simulink model "FinalSimuLab6"  (R2018b)
settings: Solver=VariableStepAuto  StartTime=0.0  StopTime=100.0  RelTol=1e-3
values from neighbouring files (symbols this model uses):
  A1 = k1    (= 8)    [FinalLab6.m]    (also in lab6.m = 2)
  a1 = Aw1*sqrt(2*g*h1max)/h1max    [FinalLab6.m]    (also in lab6.m = Aw1*sqrt(2*g*hm1)/hm1)
  A2 = k1    (= 8)    [FinalLab6.m]    (also in lab6.m = 2)
  a2 = Aw2*sqrt(2*g*h2max)/h2max    [FinalLab6.m]    (also in lab6.m = Aw2*sqrt(2*g*hm2)/hm2)
  dfwe1 = 0.1 * fwe1max    [FinalLab6.m]
  dt = 20    [FinalLab6.m]    (also in lab6.m = 10)
  fwe1 = fwe10(i)    [FinalLab6.m]    (also in lab6.m)
  fwe2 = 0    [FinalLab6.m]    (also in lab6.m)
  h10 = (fwe1 / a1) + h20    [FinalLab6.m]    (also in lab6.m = (fwe1+a1*h20)/a1)
  h20 = (fwe1 + fwe2)/a2    [FinalLab6.m]    (also in lab6.m = (fwe2+fwe1)/a2)
settings Model: Creator=wojciechkonury  LastModifiedBy=wojciechkonury

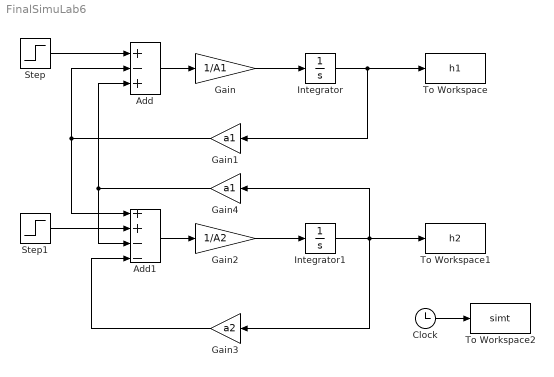
== system FinalSimuLab6 ==
  Add : Sum  Inputs=+-+
  Add1 : Sum  Inputs=++--
  Clock : Clock
  Gain : Gain  Gain=1/A1
  Gain1 : Gain  Gain=a1
  Gain2 : Gain  Gain=1/A2
  Gain3 : Gain  Gain=a2
  Gain4 : Gain  Gain=a1
  Integrator : Integrator  InitialCondition=h10
  Integrator1 : Integrator  InitialCondition=h20
  Step : Step  Time=dt  Before=fwe1  After=fwe1+dfwe1  SampleTime=0
  Step1 : Step  Time=dt  Before=fwe2  After=fwe2  SampleTime=0
  To Workspace : ToWorkspace  VariableName=h1  SampleTime=-1
  To Workspace1 : ToWorkspace  VariableName=h2  SampleTime=-1
  To Workspace2 : ToWorkspace  VariableName=simt  SampleTime=-1
  wires:
  Step/1 -> Add/1
  Add/1 -> Gain/1
  Gain/1 -> Integrator/1
  Integrator/1 -> To Workspace/1, Gain1/1
  Gain1/1 -> Add1/1, Add/2
  Step1/1 -> Add1/2
  Add1/1 -> Gain2/1
  Gain2/1 -> Integrator1/1
  Integrator1/1 -> Gain4/1, Gain3/1, To Workspace1/1
  Gain3/1 -> Add1/4
  Gain4/1 -> Add1/3, Add/3
  Clock/1 -> To Workspace2/1
